simulink model "Ejercicio_3_d"  (R2023a)
settings: Solver=VariableStepAuto  StartTime=0.0  StopTime=5  RelTol=1e-3
values from neighbouring files (symbols this model uses):
  A = [0 1; -k/m 0]    [Ejercicio_3.m]
  A_est = A - Ke*C    [Ejercicio_3.m]
  B = [0; 1/m]    [Ejercicio_3.m]
  B_est = [B Ke]    [Ejercicio_3.m]
  C_est = eye(2)    [Ejercicio_3.m]
  D_est = [0 0;0 0]'    [Ejercicio_3.m]
  g0 = utilsMati.realim_VE.factorEscala(A,B,C,K)    [Ejercicio_3.m]
  K = 2    [Ejercicio_2.m]    (also in Ejercicio_3.m = acker(A, B, PLC_VE))
settings Model: Creator=Mati  LastModifiedBy=Mati

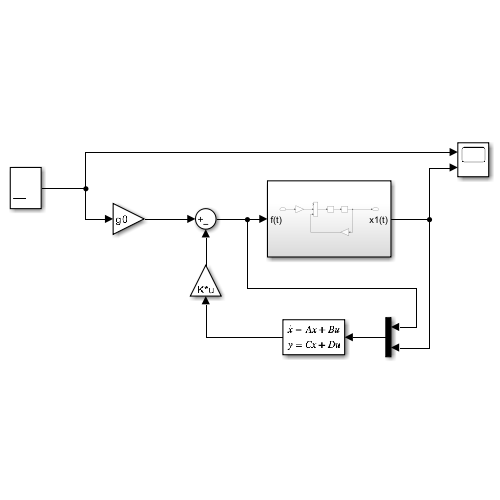
[thumbnail: Simulink's stored preview of the top-level diagram]
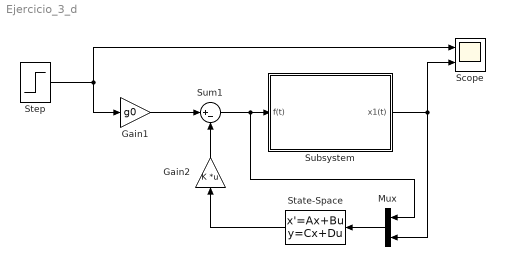
== system Ejercicio_3_d ==
  Gain1 : Gain  Gain=g0
  Gain2 : Gain  Gain=K  Multiplication=Matrix(K*u)
  Mux : Mux  Inputs=2
  Scope : Scope  NumInputPorts=2
  State-Space : StateSpace  A=A_est  B=B_est  C=C_est  D=D_est  InitialCondition=0
  Step : Step  SampleTime=0
  Subsystem : Subsystem
  Sum1 : Sum  Inputs=|+-
  wires:
  Sum1/1 -> Mux/1, Subsystem/1(f(t))
  Subsystem/1(x1(t)) -> Mux/2, Scope/2
  Step/1 -> Scope/1, Gain1/1
  Gain1/1 -> Sum1/1
  Gain2/1 -> Sum1/2
  State-Space/1 -> Gain2/1
  Mux/1 -> State-Space/1

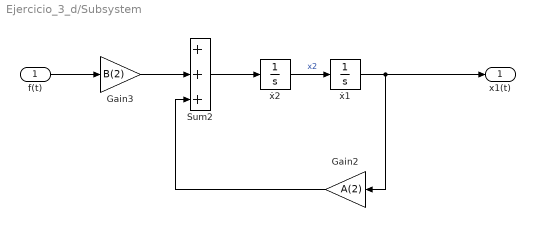
== system Ejercicio_3_d/Subsystem ==
  f(t) : Inport
  Gain2 : Gain  Gain=A(2)
  Gain3 : Gain  Gain=B(2)
  Sum2 : Sum  Inputs=+++
  ẋ1 : Integrator
  ẋ2 : Integrator
  x1(t) : Outport
  wires:
  ẋ2/1 -> ẋ1/1  "x2"
  ẋ1/1 -> x1(t)/1, Gain2/1
  f(t)/1 -> Gain3/1
  Gain3/1 -> Sum2/2
  Gain2/1 -> Sum2/3
  Sum2/1 -> ẋ2/1
